simulink model "task10"  (R2017b)
settings: Solver=VariableStepAuto  StartTime=0.0  StopTime=10.0  RelTol=1e-3
values from neighbouring files (symbols this model uses):
  A1 = [0 1 0 0;-(k1+k2)/m 0 (l1*k1-l2*k2)/m 0; 0 0 0 1;-(l1*k1-l2*k2)/J 0 -(k1*l1^2+k2*l2^2)/J 0]    [H_inf_ctrl.m]    (also in Task8.m)
  B1 = [0 0 0 0;k1/m k2/m 1/m 1/m;0 0 0 0;-k1*l1/J k2*l2/J -l1/J l2/J]    [H_inf_ctrl.m]    (also in Task8.m)
  C1 = eye(4)    [H_inf_ctrl.m]    (also in Task8.m)
  D1 = zeros(4)    [H_inf_ctrl.m]    (also in Task8.m)
  f = 8    [H_inf_ctrl.m]    (also in Task6.m = 2; Task8.m; task5.m = 0.5)
  src = 1    [H_inf_ctrl.m]    (also in Task3.m = 3; Task6.m = 3; Task8.m)
undefined symbols (not defined in the file or in its folder): Ainf, Binf, Cinf, Dinf, sigbuilder_block
settings Model: Creator=Dell  LastModifiedBy=Dell

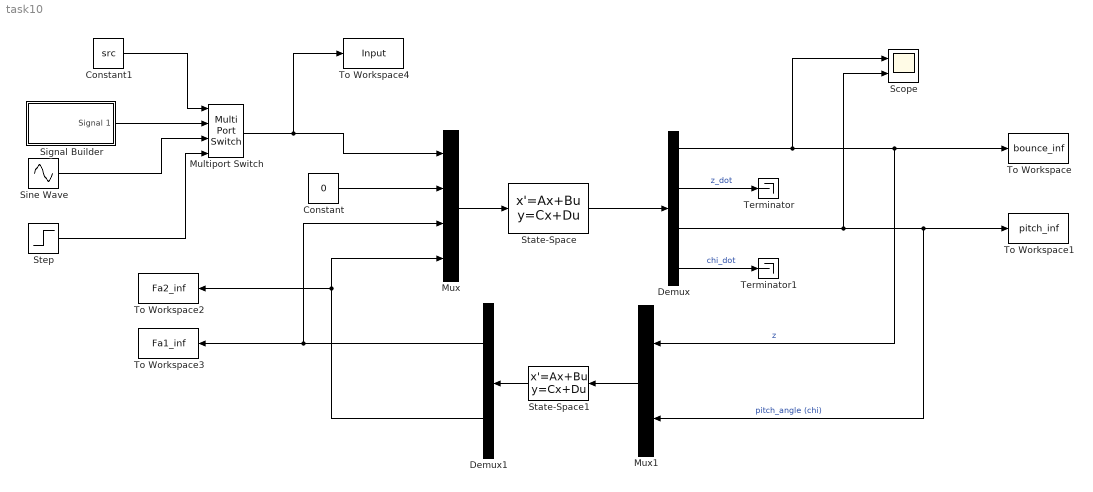
== system task10 ==
  Constant : Constant  Value=0
  Constant1 : Constant  Value=src
  Demux : Demux
  Demux1 : Demux  Outputs=2
  Multiport Switch : MultiPortSwitch
  Mux : Mux
  Mux1 : Mux  Inputs=2
  Scope : Scope  NumInputPorts=2
  Signal Builder : Subsystem  Tag=STV Subsys  LoadFcn=sigbuilder_block('load');  StartFcn=sigbuilder_block('start');  StopFcn=sigbuilder_block('stop');  ClipboardFcn=sigbuilder_block('clipboard');  mask(Sigbuilder block){tuvar=[0:10]}
      mask help: Simulink:masks:SigbuilderBlock_MD
      mask init:
      | if ~strcmp(get_param(bdroot(gcbh),'SimulationStatus'),'stopped') tuvar = sigbuilder_block('maskInit'); end
      settings: CopyFcn=sigbuilder_block('copy');  DeleteFcn=sigbuilder_block('delete');  ModelCloseFcn=sigbuilder_block('modelClose');  PreSaveFcn=sigbuilder_block('preSave');  PauseFcn=sigbuilder_block('pause');  ContinueFcn=sigbuilder_block('continue');  NameChangeFcn=sigbuilder_block('namechange');  OpenFcn=sigbuilder_block('open',[437.6 199.2 550.4 400 ]);  CloseFcn=sigbuilder_block('close');
      mask Display: plot(0, 0, 100, 100,[2, 2, 32, 32, 2], [68, 8, 8, 68, 68],[32, 2], [38, 38], [32, 19, 2],[53, 60, 44], [32, 17, 17, 2],[16, 16, 31, 31]);txt = getActiveGroup(gcbh);text(2, 100, txt,'verticalAlignment', 'top');
  Sine Wave : Sin  Amplitude=0.01  Frequency=2*pi*f  SampleTime=0
  State-Space : StateSpace  A=A1  B=B1  C=C1  D=D1  InitialCondition=0
  State-Space1 : StateSpace  A=Ainf  B=Binf  C=Cinf  D=Dinf  InitialCondition=0
  Step : Step  SampleTime=0
  Terminator : Terminator
  Terminator1 : Terminator
  To Workspace : ToWorkspace  VariableName=bounce_inf  SaveFormat=Timeseries  SampleTime=-1
  To Workspace1 : ToWorkspace  VariableName=pitch_inf  SaveFormat=Timeseries  SampleTime=-1
  To Workspace2 : ToWorkspace  VariableName=Fa2_inf  SaveFormat=Timeseries  SampleTime=-1
  To Workspace3 : ToWorkspace  VariableName=Fa1_inf  SaveFormat=Timeseries  SampleTime=-1
  To Workspace4 : ToWorkspace  VariableName=Input  SaveFormat=Timeseries  SampleTime=-1
  wires:
  Mux/1 -> State-Space/1
  Sine Wave/1 -> Multiport Switch/3
  Constant1/1 -> Multiport Switch/1
  Demux/1 -> Scope/1, Mux1/1, To Workspace/1  "z"
  Signal Builder/1(Signal 1) -> Multiport Switch/2
  Multiport Switch/1 -> To Workspace4/1, Mux/1
  Demux1/2 -> To Workspace2/1, Mux/4
  Demux1/1 -> To Workspace3/1, Mux/3
  Demux/3 -> Scope/2, Mux1/2, To Workspace1/1  "pitch_angle (chi)"
  Constant/1 -> Mux/2
  State-Space/1 -> Demux/1
  Step/1 -> Multiport Switch/4
  Mux1/1 -> State-Space1/1
  State-Space1/1 -> Demux1/1
  Demux/2 -> Terminator/1  "z_dot"
  Demux/4 -> Terminator1/1  "chi_dot"

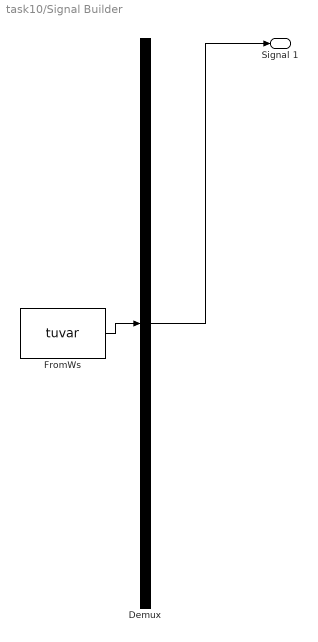
== system task10/Signal Builder ==
  Demux : Demux  Tag=STV Demux  Outputs=1
  FromWs : FromWorkspace  Tag=STV FromWs  VariableName=tuvar  SampleTime=0
      SigBuilderData=|
      | common.afterFinalStr = 'Extrapolate'
      | common.sampleTime = 0
      | dataSet.timeRange = [0 10]
      | dataSet.name = 'Group 1'
      | sbobj.Groups.Name = 'Group 1'
      | sbobj.Groups.Signals.Name = 'Signal 1'
      | sbobj.Groups.Signals.XData = [0 1 1 4.62 10]
      | sbobj.Groups.Signals.YData = [0.03 0.03 0 0 0]
  Signal 1 : Outport  Tag=STV Outport
  wires:
  Demux/1 -> Signal 1/1
  FromWs/1 -> Demux/1
